simulink model "der2023b"  (R2023b)
settings: Solver=VariableStepAuto  StartTime=0.0  StopTime=5  RelTol=1e-3
settings Model: Creator=32602  LastModifiedBy=admin
settings RTWCC: GPUComputeCapability=5.0

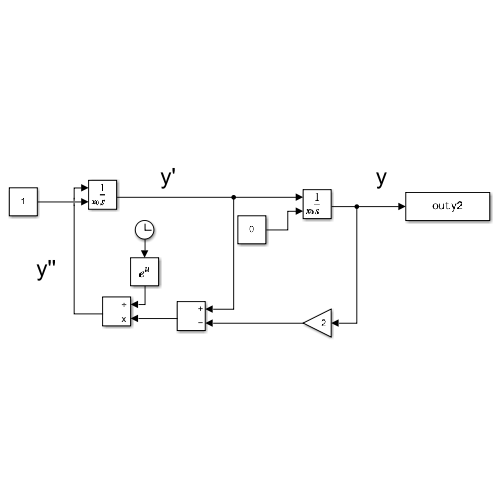
[thumbnail: Simulink's stored preview of the top-level diagram]
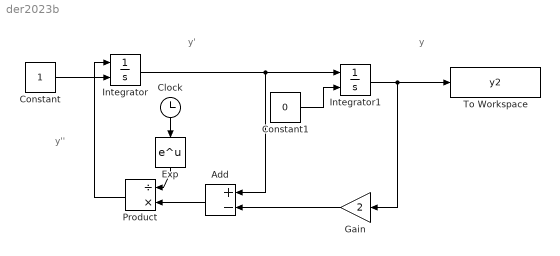
== system der2023b ==
  note: y
  note: y'
  note: y''
  Add : Sum  Inputs=+-
  Clock : Clock
  Constant : Constant
  Constant1 : Constant  Value=0
  Exp : Math
  Gain : Gain  Gain=2
  Integrator : Integrator  InitialConditionSource=external
  Integrator1 : Integrator  InitialConditionSource=external
  Product : Product  Inputs=/*
  To Workspace : ToWorkspace  VariableName=y2  SaveFormat=Timeseries  SampleTime=0.01
  wires:
  Integrator1/1 -> Gain/1, To Workspace/1
  Integrator/1 -> Integrator1/1, Add/1
  Product/1 -> Integrator/1
  Constant/1 -> Integrator/2
  Constant1/1 -> Integrator1/2
  Gain/1 -> Add/2
  Clock/1 -> Exp/1
  Exp/1 -> Product/1
  Add/1 -> Product/2
